simulink model "debug_FTExternalForces"  (Simulink 9.0)
settings: Solver=FixedStepDiscrete  StartTime=0.0  StopTime=inf  FixedStep=0.01  RelTol=1e-3  EnableMultiTasking=on
InitFcn:
  | ROBOT_DOF=23;
libraries: WBToolboxLibrary x7
settings Model: SuppressorTable=22 serialization::archive 11 0 6 0 0 0 1 0  Creator=DanielePucci  LastModifiedBy=gnava
settings DataIOCC: LimitDataPoints=on  SaveFormat=Dataset
settings DebuggingCC: UnderspecifiedInitializationDetection=Simplified  MergeDetectMultiDrivingBlocksExec=error  AllowSymbolicDim=off
settings HardwareCC: ProdBitPerPointer=64  ProdBitPerSizeT=64  ProdBitPerPtrDiffT=64  ProdLargestAtomicFloat=Float  ProdIntDivRoundTo=Zero  ProdEndianess=LittleEndian  ProdWordSize=64  ProdHWDeviceType=Intel->x86-64 (Windows64)

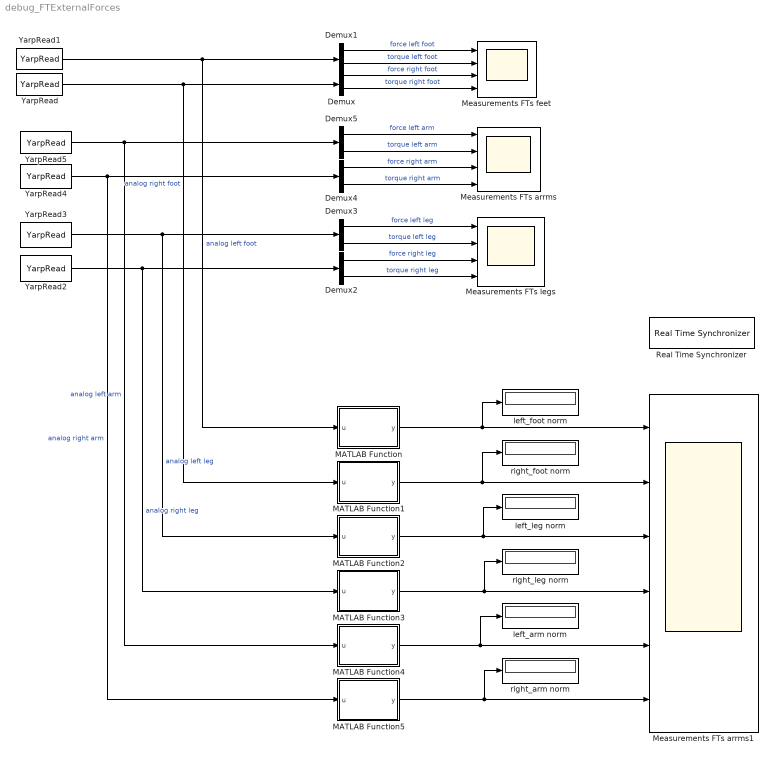
== system debug_FTExternalForces ==
  Demux{,1..5} (6 alike) : Demux  Outputs=2
  MATLAB Function : MATLAB Function  TreatAsAtomicUnit=on
  MATLAB Function1 : MATLAB Function  TreatAsAtomicUnit=on
  MATLAB Function2 : MATLAB Function  TreatAsAtomicUnit=on
  MATLAB Function3 : MATLAB Function  TreatAsAtomicUnit=on
  MATLAB Function4 : MATLAB Function  TreatAsAtomicUnit=on
  MATLAB Function5 : MATLAB Function  TreatAsAtomicUnit=on
  Measurements FTs arrms : Scope  NumInputPorts=4
  Measurements FTs arrms1 : Scope  NumInputPorts=6
  Measurements FTs feet : Scope  NumInputPorts=4
  Measurements FTs legs : Scope  NumInputPorts=4
  Real Time Synchronizer : WBToolboxLibrary/Utilities/Real Time Synchronizer  period=0.01
      settings: SourceProductName=WholeBodyToolbox
  YarpRead : WBToolboxLibrary/Utilities/YarpRead  portName='/icub/right_foot/analog:o'  signalSize=6  timeout=0.5  blocking=off  timestamp=off  autoconnect=on  errorOnConnection=off
      settings: SourceProductName=WholeBodyToolbox
  YarpRead1 : WBToolboxLibrary/Utilities/YarpRead  portName='/icub/left_foot/analog:o'  signalSize=6  timeout=0.5  blocking=off  timestamp=off  autoconnect=on  errorOnConnection=off
      settings: SourceProductName=WholeBodyToolbox
  YarpRead2 : WBToolboxLibrary/Utilities/YarpRead  portName='/icub/right_leg/analog:o'  signalSize=6  timeout=0.5  blocking=off  timestamp=off  autoconnect=on  errorOnConnection=off
      settings: SourceProductName=WholeBodyToolbox
  YarpRead3 : WBToolboxLibrary/Utilities/YarpRead  portName='/icub/left_leg/analog:o'  signalSize=6  timeout=0.5  blocking=off  timestamp=off  autoconnect=on  errorOnConnection=off
      settings: SourceProductName=WholeBodyToolbox
  YarpRead4 : WBToolboxLibrary/Utilities/YarpRead  portName='/icub/right_arm/analog:o'  signalSize=6  timeout=0.5  blocking=off  timestamp=off  autoconnect=on  errorOnConnection=off
      settings: SourceProductName=WholeBodyToolbox
  YarpRead5 : WBToolboxLibrary/Utilities/YarpRead  portName='/icub/left_arm/analog:o'  signalSize=6  timeout=0.5  blocking=off  timestamp=off  autoconnect=on  errorOnConnection=off
      settings: SourceProductName=WholeBodyToolbox
  left_arm norm : Display
  left_foot norm : Display
  left_leg norm : Display
  right_arm norm : Display
  right_foot norm : Display
  right_leg norm : Display
  wires:
  YarpRead/1 -> MATLAB Function1/1(u), Demux/1  "analog right foot"
  Demux/1 -> Measurements FTs feet/3  "force right foot"
  Demux/2 -> Measurements FTs feet/4  "torque right foot"
  YarpRead1/1 -> Demux1/1, MATLAB Function/1(u)  "analog left foot"
  Demux1/1 -> Measurements FTs feet/1  "force left foot"
  Demux1/2 -> Measurements FTs feet/2  "torque left foot"
  YarpRead2/1 -> MATLAB Function3/1(u), Demux2/1  "analog right leg"
  Demux2/1 -> Measurements FTs legs/3  "force right leg"
  Demux2/2 -> Measurements FTs legs/4  "torque right leg"
  YarpRead3/1 -> MATLAB Function2/1(u), Demux3/1  "analog left leg"
  Demux3/1 -> Measurements FTs legs/1  "force left leg"
  Demux3/2 -> Measurements FTs legs/2  "torque left leg"
  YarpRead4/1 -> MATLAB Function5/1(u), Demux4/1  "analog right arm"
  Demux4/1 -> Measurements FTs arrms/3  "force right arm"
  Demux4/2 -> Measurements FTs arrms/4  "torque right arm"
  YarpRead5/1 -> MATLAB Function4/1(u), Demux5/1  "analog left arm"
  Demux5/1 -> Measurements FTs arrms/1  "force left arm"
  Demux5/2 -> Measurements FTs arrms/2  "torque left arm"
  MATLAB Function1/1(y) -> right_foot norm/1, Measurements FTs arrms1/2
  MATLAB Function2/1(y) -> left_leg norm/1, Measurements FTs arrms1/3
  MATLAB Function3/1(y) -> right_leg norm/1, Measurements FTs arrms1/4
  MATLAB Function4/1(y) -> left_arm norm/1, Measurements FTs arrms1/5
  MATLAB Function5/1(y) -> right_arm norm/1, Measurements FTs arrms1/6
  MATLAB Function/1(y) -> left_foot norm/1, Measurements FTs arrms1/1

== matlab function MATLAB Function1 ==
  data: u input double; y output double
function y = normFCN(u)

    y = norm(u);
end

== matlab function MATLAB Function ==
  data: u input double; y output double
function y = normFCN(u)

    y = norm(u);
end

== matlab function MATLAB Function2 ==
  data: u input double; y output double
function y = normFCN(u)

    y = norm(u);
end

== matlab function MATLAB Function3 ==
  data: u input double; y output double
function y = normFCN(u)

    y = norm(u);
end

== matlab function MATLAB Function4 ==
  data: u input double; y output double
function y = normFCN(u)

    y = norm(u);
end

== matlab function MATLAB Function5 ==
  data: u input double; y output double
function y = normFCN(u)

    y = norm(u);
end
